simulink model "Galvo_sys_Cdisc_Pcont_cc_v64_proto_v13_OFFSETS_MODEL_PT1"  (R2013a)
settings: Solver=ode3  StartTime=0.0  StopTime=1e-3  FixedStep=TS  MaxStep=1e-5  RelTol=1e-3  AbsTol=1e-5
PreLoadFcn:
  | vname=@(x) inputname(1);
  | paramCtrl=evalin('base','paramCtrl;');
  | I_LIM=str2num(paramCtrl.I_LIM);
  | Kbc=str2num(paramCtrl.Kbc);
  | FS=evalin('base','FS;');
InitFcn:
  | %%%%%%  set scope time range
  | T_STOP=str2num(get_param(gcs,'StopTime'));
  | if numel(T_STOP) > 1
  |    T_STOP=T_STOP(2);
  | else
  |    T_STOP=T_STOP(1);
  | end
  | T_STOP=num2str(T_STOP);
  | 
  | %%%%%%  set scope time range in system @init_callback_fct
  | T_STOP=num2str(str2num(get_param(gcs,'StopTime')));
  | 
  | childs = allchild(0);
  | sol=strfind(upper(get(allchild(0),'Tag')),'VIEWER_PARAMETERS');
  | 
  | if iscell(sol)
  |    ind=find(~cellfun(@isempty, strfind(upper(get(allchild(0),'Tag')),'VIEWER_PARAMETERS')));
  | else
  |    ind=sol;
  | end
  | %ind=find(~cellfun(@isempty, {strfind(upper(get(allchild(0),'Tag')),'VIEWER_PARAMETERS'),[]}))
  | if ~isempty(ind)
  |    for k=1:length(childs(ind))
  |       set_param(getfield(get(childs(ind(k)),'UserData'),'block'),'TimeRange',T_STOP);
  |       get_param(getfield(get(childs(ind(k)),'UserData'),'block'),'TimeRange');
  | %    set_param(getfield(get(childs(ind),'UserData'),'block'),'TimeRange',T_STOP);
  | %    get_param(getfield(get(childs(ind),'UserData'),'block'),'TimeRange');
  |    end
  | else
  |     warning(sprintf('VIEWER_PARAMETERS object not found\nOpen the config dialog by hand for the first sim start'))
  | end
StartFcn:
  | I_LIM=str2num(paramCtrl.I_LIM);
  | Kbc=str2num(paramCtrl.Kbc);
  | %FS=evalin('base','FS;');
undefined symbols (not defined in the file or in its folder): LSB, TS
libraries: simulink_extras x1, simulink x1
settings Model: BufferReuse=off  Creator=mainster  LastModifiedBy=mainster
settings SolverCC: AutoInsertRateTranBlk=on
settings DataIOCC: LimitDataPoints=off  SaveOutput=off  SaveTime=off
settings OptimizationCC: BlockReduction=off  InlineParams=on  OptimizeBlockIOStorage=off  BufferReuse=off  ExpressionFolding=off  LocalBlockOutputs=off
settings DebuggingCC: ArtificialAlgebraicLoopMsg=none  InitInArrayFormatMsg=none  LoggingUnavailableSignals=none
settings HardwareCC: ProdLargestAtomicInteger=Long  ProdLargestAtomicFloat=Double  ProdEndianess=LittleEndian  ProdHWDeviceType=ARM Compatible->ARM Cortex
settings ModelReferenceCC: ModelReferenceNumInstancesAllowed=Single

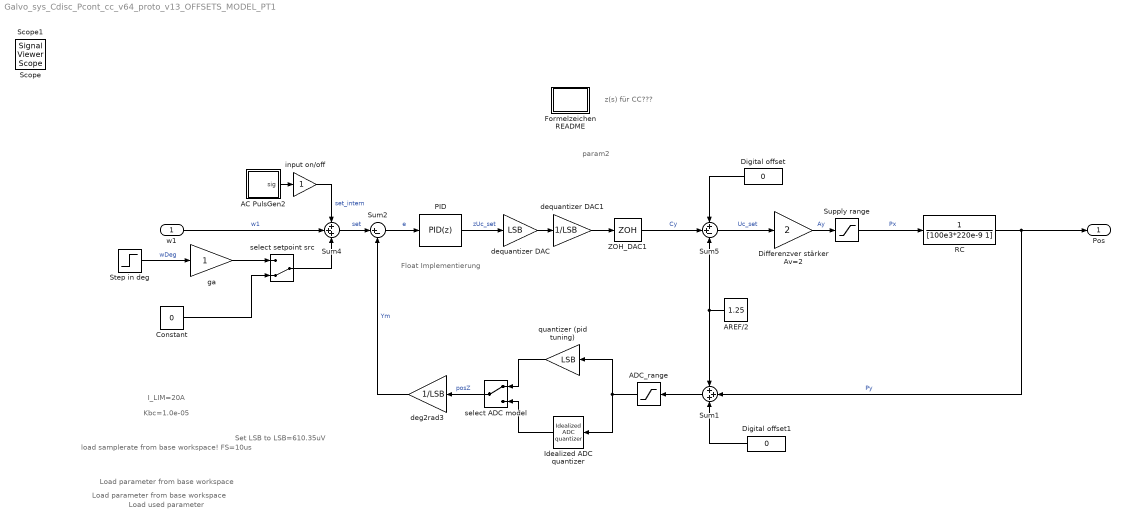
== system Galvo_sys_Cdisc_Pcont_cc_v64_proto_v13_OFFSETS_MODEL_PT1 ==
  note: Float
      | Implementierung
  note: z(s) für
      | CC???
  note: param2
  note: I_LIM=20A
  note: Kbc=1.0e-05
  note: load samplerate from
      | base workspace!
      | FS=10us
  note: Load parameter from
      | base workspace
  note: Load used parameter
  note: Load parameter from
      | base workspace
  note: Set LSB to
      | LSB=610.35uV
  w1 : Inport
  AC PulsGen2 : Subsystem  mask{sigp=1, sigpp=0, offs=0}
      mask prompts: sigp "Insert signal peak"; sigpp "or signal peak-to-peak"; offs "Insert DC offset"
      mask TypeOptions sigp: PulsGen/Amplitude
      mask Callback sigp:
      | %sigp=get_param([gcb '/PulsGen'],'Amplitude')
      | %SigVal=2*sigp
      mask TypeOptions offs: offset/Value
      mask Display:
      | %str=sprintf('%s',get(gcbh,'ModelName'));
      | port_label('output', 1, '','texmode','off')
      | %text(.05,.98,['{\fontsize{12}\it\bf' strrep(str,'_',' ') '}'],'horizontalAlignment','left','verticalAlignment','top','texmode','on')
      | %text(.5,0.95,['{\fontsize{8}A_{peak}=}'],'horizontalAlignment','center','verticalAlignment','top','texmode','on')
      | disp(sprintf('Up=%.3g\nDC=%.3g',sigp, offs))
      | %disp(['Upp=' sigpp])%, offs))
      | %sprintf('sigpp==%s',sigpp)
      | %text(.15,.05,['{\fontsize{10}\itmechanics}'],'horizontalAlignment','left','verticalAlignment','bottom','texmode','on')
  ADC_range : Saturate  UpperLimit=2.5  LowerLimit=0
      settings: AttributesFormatString=V_min=%<UpperLimit>\nV_max=%<LowerLimit>
  AREF/2 : Constant  Value=1.25  SampleTime=-1
  Constant : Constant  Value=0  SampleTime=TS
  Differenzver stärker Av=2 : Gain  Gain=2
  Digital offset : Constant  Value=0  SampleTime=TS
  Digital offset1 : Constant  Value=0  SampleTime=TS
  Formelzeichen README : Subsystem
  Idealized ADC quantizer : simulink_extras/Additional Discrete/Idealized ADC quantizer  NumberOfConverterBits=12  Vmin=0  Vmax=2.5  OutputDataType=uint16  OutputNegativeValues=off
  PID : simulink/Continuous/PID Controller  Controller=PID  TimeDomain=Discrete-time  SampleTime=TS  IntegratorMethod=Forward Euler  FilterMethod=Forward Euler  Form=Parallel  P=406.220491913229  I=112878.065273991  D=-0.00567196917468385  N=36769.7002550283  InitialConditionSource=internal  InitialConditionForIntegrator=0  InitialConditionForFilter=0  ExternalReset=none  IgnoreLimit=on  LimitOutput=on  UpperSaturationLimit=1.25  LowerSaturationLimit=-1.25  LinearizeAsGain=on  AntiWindupMode=clamping  Kb=0.1  TrackingMode=off  Kt=0  PParamMin=[]  PParamMax=[]  PParamDataTypeStr=double  IParamMin=[]  IParamMax=[]  IParamDataTypeStr=double  DParamMin=[]  DParamMax=[]  DParamDataTypeStr=double  NParamMin=[]  NParamMax=[]  KbParamMin=[]  KbParamMax=[]  KtParamMin=[]  KtParamMax=[]  POutMin=[]  POutMax=[]  IOutMin=[]  IOutMax=[]  DOutMin=[]  DOutMax=[]  NOutMin=[]  NOutMax=[]  KbOutMin=[]  KbOutMax=[]  KtOutMin=[]  KtOutMax=[]  IntegratorOutMin=[]  IntegratorOutMax=[]  FilterOutMin=[]  FilterOutMax=[]  SumOutMin=[]  SumOutMax=[]  SumI1OutMin=[]  SumI1OutMax=[]  SumI2OutMin=[]  SumI2OutMax=[]  SumI3OutMin=[]  SumI3OutMax=[]  SumDOutMin=[]  SumDOutMax=[]  SaturationOutMin=[]  SaturationOutMax=[]  IntegratorContinuousStateAttributes=''  IntegratorStateMustResolveToSignalObject=off  IntegratorRTWStateStorageClass=Auto  FilterContinuousStateAttributes=''  FilterStateMustResolveToSignalObject=off  FilterRTWStateStorageClass=Auto
      settings: AttributesFormatString=Kp: %<P>\nKi: %<I>\nKd: %<D>\nuplim: %<UpperSaturationLimit>\nlolim: %<LowerSaturationLimit>
  RC : TransferFcn  Denominator=[100e3*220e-9 1]
  Step in deg : Step  Time=1e-3  SampleTime=TS  ZeroCross=off
      settings: AttributesFormatString=Ampl.: %<After>\ntime:%<Time>
  Sum1 : Sum  Inputs=+++
  Sum2 : Sum  Inputs=|+-
  Sum4 : Sum  Inputs=+++  SampleTime=TS
  Sum5 : Sum  Inputs=++-
  Supply range : Saturate  UpperLimit=2.35  LowerLimit=-2.35
      settings: AttributesFormatString=V_min=%<UpperLimit>\nV_max=%<LowerLimit>
  ZOH_DAC1 : ZeroOrderHold  SampleTime=-1
      settings: AttributesFormatString=Ts=%<SampleTime>
  deg2rad3 : Gain  Gain=1/LSB
  dequantizer DAC : Gain  Gain=LSB
  dequantizer DAC1 : Gain  Gain=1/LSB
  ga : Gain
  input on/off : Gain
  quantizer (pid tuning) : Gain  Gain=LSB
  select ADC model : ManualSwitch
  select setpoint src : ManualSwitch  CurrentSetting=0
  Pos : Outport
  Scope : SignalViewerScope  IOType=viewer  NumInputPorts=5  RefreshTime=0.033391
      settings: ShowLegends=on  TimeRange=0.001  YMin=-1~-2~-1.5~-3~-2.5  YMax=2~2~1.5~2~0.5
  Scope1 : SignalViewerScope  IOType=viewer  NumInputPorts=5  RefreshTime=0.035000
      settings: ShowLegends=on  TimeRange=0.025  YMin=-10~0~-0.5~-20~0  YMax=10~1.5~1~30~120
  wires:
  w1/1 -> Sum4/2  "w1"
  AC PulsGen2/1(sig) -> input on/off/1
  Sum2/1 -> PID/1  "e"
  Sum4/1 -> Sum2/1  "set"
  Step in deg/1 -> ga/1  "wDeg"
  input on/off/1 -> Sum4/1  "set_intern"
  PID/1 -> dequantizer DAC/1  "zUc_set"
  RC/1 -> Sum1/2, Pos/1  "Py"
  ZOH_DAC1/1 -> Sum5/2  "Cy"
  select setpoint src/1 -> Sum4/3
  deg2rad3/1 -> Sum2/2  "Ym"
  ga/1 -> select setpoint src/1
  dequantizer DAC/1 -> dequantizer DAC1/1
  Sum5/1 -> Differenzver stärker Av=2/1  "Uc_set"
  quantizer (pid tuning)/1 -> select ADC model/1
  Idealized ADC quantizer/1 -> select ADC model/2
  ADC_range/1 -> quantizer (pid tuning)/1, Idealized ADC quantizer/1
  Sum1/1 -> ADC_range/1
  Constant/1 -> select setpoint src/2
  dequantizer DAC1/1 -> ZOH_DAC1/1
  Digital offset/1 -> Sum5/1
  Digital offset1/1 -> Sum1/3
  Differenzver stärker Av=2/1 -> Supply range/1  "Ay"
  AREF/2/1 -> Sum1/1, Sum5/3
  select ADC model/1 -> deg2rad3/1  "posZ"
  Supply range/1 -> RC/1  "Px"

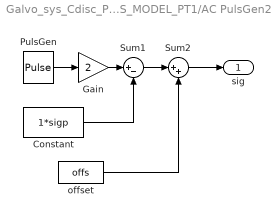
== system Galvo_sys_Cdisc_Pcont_cc_v64_proto_v13_OFFSETS_MODEL_PT1/AC PulsGen2 ==
  Constant : Constant  Value=1*sigp  SampleTime=TS
  Gain : Gain  Gain=2  SampleTime=TS
  PulsGen : DiscretePulseGenerator  Amplitude=sigp  Period=500  PulseWidth=250  SampleTime=TS
      settings: AttributesFormatString=A=%<Amplitude>\nPeri=%<Period>
  Sum1 : Sum  Inputs=|+-  SampleTime=TS
  Sum2 : Sum  Inputs=|++  SampleTime=TS
  offset : Constant  Value=offs  SampleTime=TS
  sig : Outport
  wires:
  Sum2/1 -> sig/1
  PulsGen/1 -> Gain/1
  offset/1 -> Sum2/2
  Gain/1 -> Sum1/1
  Sum1/1 -> Sum2/1
  Constant/1 -> Sum1/2

== system Galvo_sys_Cdisc_Pcont_cc_v64_proto_v13_OFFSETS_MODEL_PT1/Formelzeichen README ==
  note: Te: 		electrical torque, gen. by coils		[Nm]
      |  Ic: 			coil current							[A]
      |  Tfr:		rotor dynamic friction torque 		[Nm]
      |  Trb:		torsion bar torque					[Nm]
      |  Tw:		angular momentum				[Nm*s]
      |  w:			angular velocity 					[rad/s]
      |  yrad:		angular position 					[rad]
      |  ydeg:		angular position 					[°]
      |  Ucci:		current controller input				[V]
      |  Ucco:		current controller output			[V]
      |  Ush:		shunt voltage						[V]
  note: L_{c  }	coil inductance 							[H]
      |  R_{c  }	coil resistance							[\Omega]
      |  R_{SH }	current shunt resistance				[\Omega]
      |  J_{R  }	rotor inertia 							[kg*m²]
      |  K_{TB }	torsion bar torque const. 			[Nm/rad]
      |  K_{BM }	back EMF const.							[V*s/rad]
      |  K_{FR }	rotor dyn. friction torque const.	[Nm*s/rad]
      |  K_{MT }	el. magnetic torque const.			[Nm/A]
  note: balance of force: 	Te=Ttb+Tfr
      | 					Te - (Ttb+Tfr)=0  ->  no movement
      |
      |  integrate( 1 Nm )dt = 1 Nm*s
      |  (Nm*s)(kg*m²)⁻¹ = (N*s/kg)*m⁻¹ = m/(s*m) = rad
  note: prototyp v1.3
      | 28-04-2015
      |
      | Signal + Power PCB
      | * Allgemeine überprüfung des Regleralgorithmus
      | * Galvo #1 an Endstufe, DAC channel 1 (setI_x)
      | * pos. feedback über ADC Y weil bei ADC X der SAR-Treiber kaputt ist
      | * Parametrierung des diskreten PID Galvo Qt Gui während Laufzeit
      |
      | * Stimmen Matlab Parameter mit reel verwendeten parametern
      |   wenigstens ansatzweise überein???
